simulink model "ExampleBoundingBox"  (Simulink 9.2)
settings: Solver=FixedStepDiscrete  StartTime=0.0  StopTime=inf  FixedStep=0.001  RelTol=1e-3  EnableMultiTasking=on
libraries: rFproPhysicsLib x4
settings Model: Creator=enewton  LastModifiedBy=SeanKavanagh
settings DataIOCC: SaveOutput=off  SaveTime=off
settings OptimizationCC: ExpressionDepthLimit=2147483647  EfficientFloat2IntCast=on
settings DebuggingCC: SolverPrmCheckMsg=warning
settings RTWCC: SystemTargetFile=rfpro.tlc  MakeCommand="make_rtw OPTS=\"-DRUN_PHYSICS\""  TemplateMakefile=rfpro.tmf  Description=rFpro Target (Run Physics)  TargetLang=C++
settings STFCustomTargetCC: ModelReferenceCompliant=off  GeneratePreprocessorConditionals=Disable all  CombineOutputUpdateFcns=on  MatFileLogging=on  CPPClassGenCompliant=on  GRTInterface=off  SystemTargetFile=rfpro.tlc
settings GRTTargetCC: ModelReferenceCompliant=off  ParMdlRefBuildCompliant=off  CompOptLevelCompliant=off  ConcurrentExecutionCompliant=off  CombineOutputUpdateFcns=on  GRTInterface=off  UseToolchainInfoCompliant=off

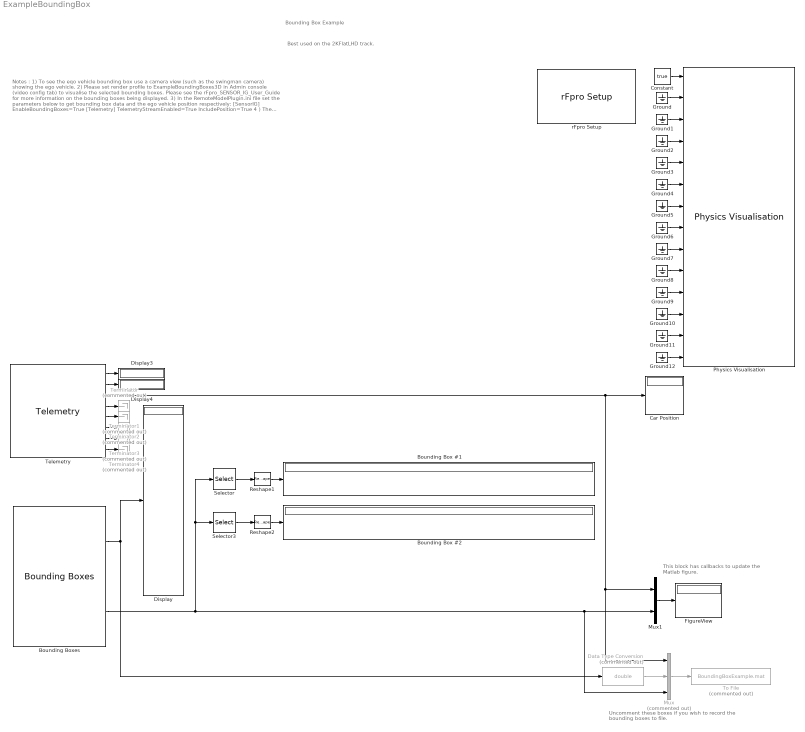
== system ExampleBoundingBox ==
  note: This block has callbacks to
      | update the Matlab figure.
  note: Uncomment these boxes if you wish to
      | record the bounding boxes to file.
  note: Bounding Box Example
  note: Notes :
      |
      | 1) To see the eqo vehicle bounding box use a camera view (such as the swingman camera)
      | showing the ego vehicle.
      |
      | 2) Please set render profile to ExampleBoundingBoxes3D in Admin console (video config tab)
      | to visualise the selected bounding boxes. Please see the rFpro_SENSOR_IG_User_Guide for more
      | information on the bounding boxes being displayed.
      |
      | 3) In the RemoteModelPlugin.ini file set the parameters below to get bounding box data and the ego
      | vehicle position respectively:
      |
      | [SensorIG]
      | EnableBoundingBoxes=True
      |
      | [Telemetry]
      | TelemetryStreamEnabled=True
      | IncludePosition=True
      |
      | 4 ) The "FigureView" block (in light blue) will display a Matlab figure with visible bounding boxes displayed in both a
      | global view and a near view. This makes use of the "ExampleBoundingBoxUpdate" script in the library folder.
      |
      | The global view will have a grey box at the position of the ego vehlcle for reference while the near view is centered on
      | the ego vehicle position - as long as the ego telemetry stream is active (see point 3 above).
      |
      | 5) Bounding boxes are limited (in the mask of the bounding box block) to those whose names match:
      | {'SLOT*', 'SP*', 'RM*', 'TL*'}
      | To see all the bounding boxes possible change this to {'*'}.
  note: Best used on the 2KFlatLHD track.
  Bounding Box #1 : Display
  Bounding Box #2 : Display
  Bounding Boxes : rFproPhysicsLib/Bounding Boxes  names={'SLOT*', 'SP*', 'RM*', 'TL*'}  groupId=0  numBoxes=19  byteStr=[]  useReverseByteOrder=off  rFpro__platform=Remote Model - Default
  Car Position : Display
  Constant : Constant  Value=true
  Data Type Conversion : DataTypeConversion  Commented=on  OutDataTypeStr=double
  Display : Display
  Display3 : Display
  Display4 : Display
  FigureView : Display
      settings: StopFcn=clear fig_listener
      settings: StartFcn=|
      | figure(1)
      | clf
      | subplot(2,1,1)
      | axis equal
      | axis([-300 300 -300 300 -10 10])
      | view(3)
      | title('Global view')
      | xlabel('X Axis');
      | ylabel('Y Axis');
      | grid
      | 
      | numBox = 19;
      | pinfo.Vertices = [0,0,0; 0,0,1; 0,1,1; 0,1,0; 1,0,0; 1,0,1; 1,1,1; 1,1,0];
      | pinfo.Faces = [1 2 3 4; 1 2 6 5; 1 4 8 5; 7 3 2 6; 7 3 4 8; 7 6 5 8];
      | pinfo.FaceAlpha = 0.1;
      | 
      | pinfo.FaceColor = 'k';
      | egoBox = patch(pinfo);
      | 
      | boxPlotGlobal = zeros(numBox, 1);
      | for iter = 0:(numBox-1)
      |   frac = iter/(numBox-1);
      |   pinfo.FaceColor = [1-frac, 0, frac];
      |   boxPlotGlobal(iter+1) = patch(pinfo);
      | end
      | 
      | subplot(2,1,2)
      | axis equal
      | axis([-50 50 -50 50 -10 10])
      | view(3)
      | title('Near view')
      | xlabel('X Axis');
      | ylabel('Y Axis');
      | grid
      | 
      | boxPlotLocal = zeros(numBox, 1);
      | for iter = 0:(numBox-1)
      |   frac = iter/(numBox-1);
      |   pinfo.FaceColor = [1-frac, 0, frac];
      |   boxPlotLocal(iter+1) = patch(pinfo);
      | end
      | 
      | clear iter numBox frac pinfo
      | 
      | fig_listener = add_exec_event_listener(gcb, 'PostOutputs', @ExampleBoundingBoxUpdate);
  Ground{,1..12} (13 alike) : Ground
  Mux : Mux  Commented=on  Inputs=3
  Mux1 : Mux  Inputs=2
  Physics Visualisation : rFproPhysicsLib/Physics Visualisation  PAR_SKIP_INTERNAL_PHYSICS=off  PAR_ACCEL_VALID=off  PAR_ROT_ACCEL_VALID=off  PAR_GEAR_VALID=off  PAR_RPM_VALID=off  PAR_INPUTS_VALID=off  PAR_STEER_TORQUE_VALID=off  PAR_HEADLIGHTS_ON_VALID=off  PAR_WHEEL_POS_VALID=off  PAR_WHEEL_ORI_VALID=off  PAR_TYRE_PARAMS_VALID=off  PAR_WHEEL_ROTATION_VALID=off  PAR_WHEEL_BRAKE_TEMP_VALID=off  PAR_WHEEL_TREAD_TEMP_VALID=off  PAR_WHEEL_AIR_TEMP_VALID=off  period=-1  offset=0  useReverseByteOrder=on  rFpro__platform=Remote Model - Default
  Reshape1 : Reshape  OutputDimensionality=Customize  OutputDimensions=[3,8]
  Reshape2 : Reshape  OutputDimensionality=Customize  OutputDimensions=[3,8]
  Selector : Selector  IndexOptions=Index vector (dialog)  Indices=[1:24]  OutputSizes=1
  Selector3 : Selector  IndexOptions=Index vector (dialog)  Indices=[25:48]  OutputSizes=1
  Telemetry : rFproPhysicsLib/Telemetry
  Terminator{,1..4} (5 alike) : Terminator  Commented=on
  To File : ToFile  Commented=on  Filename=BoundingBoxExample.mat  MatrixName=boundingBoxes
      settings: Decimation=100
  rFpro Setup : rFproPhysicsLib/rFpro Setup  platform=Remote Model - Default  stopOnSessionEnd=on  usePseudoRealtime=on  syncToRF=on  useReverseByteOrder=off  useRfTime=on  minIterations=4  maxIterations=1000  ipReceiveAddress='127.0.0.1'  ipReceivePort=11054  receiveSampleTime=-1  ipTransmitAddress='127.0.0.1'  ipTransmitPort=11052  transmitSampleTime=-1  pluginType=RUN_PHYSICS  sysTarget=xpctarget.tlc  templateMakeFile=xpc_default_tmf  makeCommand=make_rtw  buildDesc=xPC target
  wires:
  Constant/1 -> Physics Visualisation/1
  Ground/1 -> Physics Visualisation/2
  Ground1/1 -> Physics Visualisation/3
  Ground2/1 -> Physics Visualisation/4
  Ground3/1 -> Physics Visualisation/5
  Ground4/1 -> Physics Visualisation/6
  Ground5/1 -> Physics Visualisation/7
  Ground6/1 -> Physics Visualisation/8
  Ground7/1 -> Physics Visualisation/9
  Ground8/1 -> Physics Visualisation/10
  Ground9/1 -> Physics Visualisation/11
  Ground10/1 -> Physics Visualisation/12
  Ground11/1 -> Physics Visualisation/13
  Ground12/1 -> Physics Visualisation/14
  Bounding Boxes/1 -> Data Type Conversion/1, Display/1
  Telemetry/3 -> Car Position/1, Mux1/1, Mux/1
  Telemetry/1 -> Display3/1
  Telemetry/2 -> Display4/1
  Telemetry/4 -> Terminator/1
  Telemetry/5 -> Terminator1/1
  Telemetry/6 -> Terminator2/1
  Telemetry/7 -> Terminator3/1
  Telemetry/8 -> Terminator4/1
  Selector/1 -> Reshape1/1
  Reshape1/1 -> Bounding Box #1/1
  Bounding Boxes/2 -> Mux1/2, Mux/3, Selector/1, Selector3/1
  Reshape2/1 -> Bounding Box #2/1
  Selector3/1 -> Reshape2/1
  Mux/1 -> To File/1
  Data Type Conversion/1 -> Mux/2
  Mux1/1 -> FigureView/1
